simulink model "Ex_Sep_2020"  (R2022b)
settings: Solver=VariableStepAuto  StartTime=0.0  StopTime=150  RelTol=1e-3
settings Model: Creator=rrilo  LastModifiedBy=rrilo

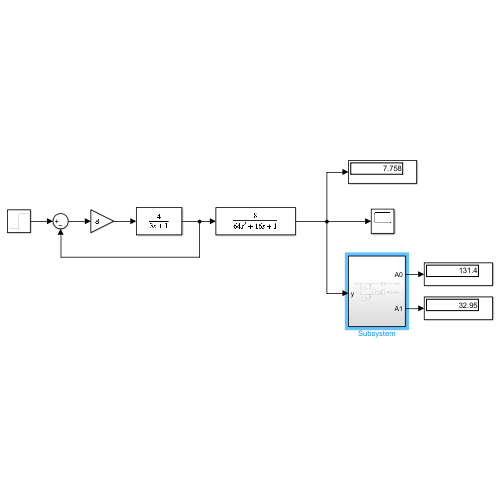
[thumbnail: Simulink's stored preview of the top-level diagram]
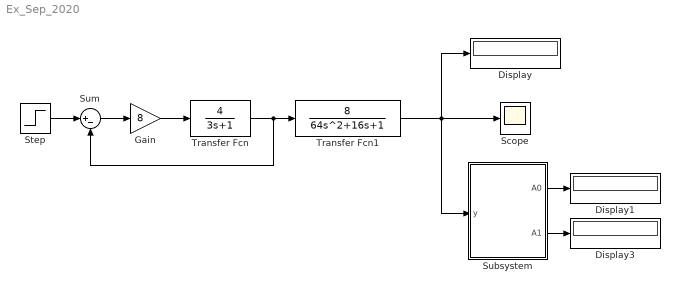
== system Ex_Sep_2020 ==
  Display : Display
  Display1 : Display
  Display3 : Display
  Gain : Gain  Gain=8
  Scope : Scope
  Step : Step  SampleTime=0
  Subsystem : Subsystem
  Sum : Sum  Inputs=|+-
  Transfer Fcn : TransferFcn  Numerator=[4]  Denominator=[3 1]
  Transfer Fcn1 : TransferFcn  Numerator=[8]  Denominator=[64 16 1]
  wires:
  Sum/1 -> Gain/1
  Step/1 -> Sum/1
  Transfer Fcn/1 -> Sum/2, Transfer Fcn1/1
  Gain/1 -> Transfer Fcn/1
  Transfer Fcn1/1 -> Subsystem/1(y), Display/1, Scope/1
  Subsystem/1(A0) -> Display1/1
  Subsystem/2(A1) -> Display3/1

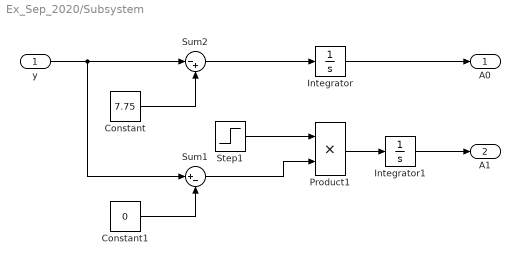
== system Ex_Sep_2020/Subsystem ==
  y : Inport
  Constant : Constant  Value=7.75
  Constant1 : Constant  Value=0
  Integrator : Integrator
  Integrator1 : Integrator
  Product1 : Product
  Step1 : Step  Time=16.95  Before=1  After=0  SampleTime=0
  Sum1 : Sum  Inputs=|+-
  Sum2 : Sum  Inputs=|-+
  A0 : Outport
  A1 : Outport  Port=2
  wires:
  y/1 -> Sum1/1, Sum2/1
  Integrator1/1 -> A1/1
  Step1/1 -> Product1/1
  Sum1/1 -> Product1/2
  Constant/1 -> Sum2/2
  Constant1/1 -> Sum1/2
  Sum2/1 -> Integrator/1
  Product1/1 -> Integrator1/1
  Integrator/1 -> A0/1
